simulink model "system_composer_test1"  (R2023b)
settings: Solver=VariableStepAuto  StartTime=0.0  StopTime=10.0  RelTol=1e-3
settings Model: Creator=jcm52  LastModifiedBy=jcm52

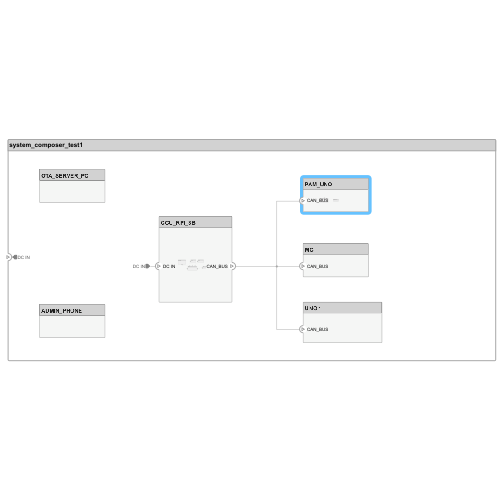
[thumbnail: Simulink's stored preview of the top-level diagram]
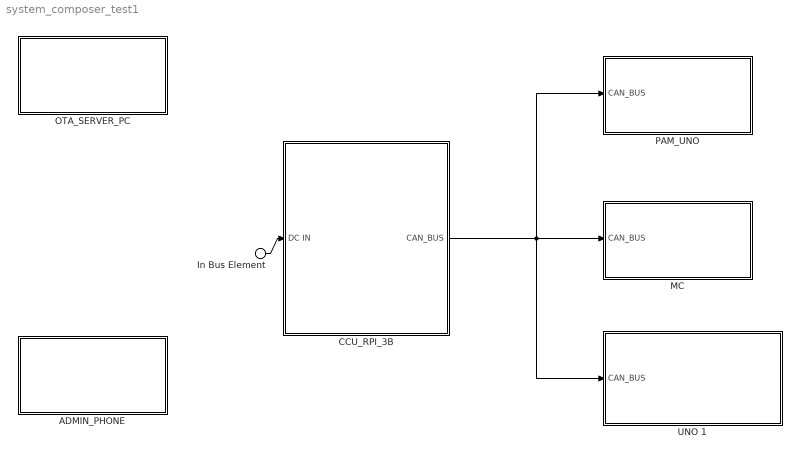
== system system_composer_test1 ==
  In Bus Element : Inport  PortName=DC IN
  ADMIN_PHONE : Subsystem
      settings: PortSchema="{\"entries\":[{\"content\":{\"headerSize\":26,\"margin\":15,\"minimumSpacing\":25,\"sides\":[{\"content\":{},\"type\":\"ConnectorPlacement.EquallySpacedRectSide\",\"uuid\":\"7e3d46c6-9eeb-4d23-9c3d-9bca39c5abc5\"},{\"content\":{\"side\":\"RIGHT\"},\"type\":\"ConnectorPlacement.EquallySpacedRectSide\",\"uuid\":\"9f2ff8fd-d14b-486f-a742-18e492795d25\"},{\"content\":{\"side\":\"TOP\"},\"type\":\"ConnectorPlacement.EquallySpacedRectSide\",\"uuid\":\"e95812f2-ccc1-4a86-ac53-e7b35601f911\"}]},\"type\":\"ConnectorPlacement.EquallySpacedConnector\",\"uuid\":\"2d0f1e9a-6af9-4d3f-b8da-a747a1ef6490\"}],\"packageUris\":[\"http://schema.mathworks.com/mf0/Connector/R2020b\"],\"version\":\"1.0\"}"
  CCU_RPI_3B : Subsystem
      settings: PortSchema="{\"entries\":[{\"content\":{\"headerSize\":26,\"margin\":15,\"minimumSpacing\":25,\"sides\":[{\"content\":{\"connectorIds\":[\"In1\"]},\"type\":\"ConnectorPlacement.EquallySpacedRectSide\",\"uuid\":\"35364ac4-dc3e-4266-bc20-925e01ca6202\"},{\"content\":{\"connectorIds\":[\"Out1\"],\"side\":\"RIGHT\"},\"type\":\"ConnectorPlacement.EquallySpacedRectSide\",\"uuid\":\"050ee6e0-40ef-4ced-bbf4-001a02d9c667\"},{\"content\":{\"side\":\"TOP\"},\"type\":\"ConnectorPlacement.EquallySpacedRectSide\",\"uuid\":\"0258bc82-266f-47dd-a28d-284b42f54e02\"},{\"content\":{\"side\":\"BOTTOM\"},\"type\":\"ConnectorPlacement.EquallySpacedRectSide\",\"uuid\":\"ceb5ff19-933f-4c7c-8606-80ebf5710174\"}]},\"type\":\"ConnectorPlacement.EquallySpacedConnector\",\"uuid\":\"a71d942b-361d-4a00-a580-c54bc0bd10ca\"}],\"packageUris\":[\"http://schema.mathworks.com/mf0/Connector/R2020b\"],\"version\":\"1.0\"}"
  MC : Subsystem
      settings: PortSchema="{\"entries\":[{\"content\":{\"headerSize\":26,\"margin\":15,\"minimumSpacing\":25,\"sides\":[{\"content\":{\"connectorIds\":[\"In1\"]},\"type\":\"ConnectorPlacement.EquallySpacedRectSide\",\"uuid\":\"35364ac4-dc3e-4266-bc20-925e01ca6202\"},{\"content\":{\"side\":\"RIGHT\"},\"type\":\"ConnectorPlacement.EquallySpacedRectSide\",\"uuid\":\"050ee6e0-40ef-4ced-bbf4-001a02d9c667\"},{\"content\":{\"side\":\"TOP\"},\"type\":\"ConnectorPlacement.EquallySpacedRectSide\",\"uuid\":\"0258bc82-266f-47dd-a28d-284b42f54e02\"}]},\"type\":\"ConnectorPlacement.EquallySpacedConnector\",\"uuid\":\"a71d942b-361d-4a00-a580-c54bc0bd10ca\"}],\"packageUris\":[\"http://schema.mathworks.com/mf0/Connector/R2020b\"],\"version\":\"1.0\"}"
  OTA_SERVER_PC : Subsystem
      settings: PortSchema="{\"entries\":[{\"content\":{\"headerSize\":26,\"margin\":15,\"minimumSpacing\":25,\"sides\":[{\"content\":{},\"type\":\"ConnectorPlacement.EquallySpacedRectSide\",\"uuid\":\"7e3d46c6-9eeb-4d23-9c3d-9bca39c5abc5\"},{\"content\":{\"side\":\"RIGHT\"},\"type\":\"ConnectorPlacement.EquallySpacedRectSide\",\"uuid\":\"9f2ff8fd-d14b-486f-a742-18e492795d25\"},{\"content\":{\"side\":\"TOP\"},\"type\":\"ConnectorPlacement.EquallySpacedRectSide\",\"uuid\":\"e95812f2-ccc1-4a86-ac53-e7b35601f911\"}]},\"type\":\"ConnectorPlacement.EquallySpacedConnector\",\"uuid\":\"2d0f1e9a-6af9-4d3f-b8da-a747a1ef6490\"}],\"packageUris\":[\"http://schema.mathworks.com/mf0/Connector/R2020b\"],\"version\":\"1.0\"}"
  PAM_UNO : Subsystem
      settings: PortSchema="{\"entries\":[{\"content\":{\"headerSize\":26,\"margin\":15,\"minimumSpacing\":25,\"sides\":[{\"content\":{\"connectorIds\":[\"In1\"]},\"type\":\"ConnectorPlacement.EquallySpacedRectSide\",\"uuid\":\"35364ac4-dc3e-4266-bc20-925e01ca6202\"},{\"content\":{\"side\":\"RIGHT\"},\"type\":\"ConnectorPlacement.EquallySpacedRectSide\",\"uuid\":\"050ee6e0-40ef-4ced-bbf4-001a02d9c667\"},{\"content\":{\"side\":\"TOP\"},\"type\":\"ConnectorPlacement.EquallySpacedRectSide\",\"uuid\":\"0258bc82-266f-47dd-a28d-284b42f54e02\"}]},\"type\":\"ConnectorPlacement.EquallySpacedConnector\",\"uuid\":\"a71d942b-361d-4a00-a580-c54bc0bd10ca\"}],\"packageUris\":[\"http://schema.mathworks.com/mf0/Connector/R2020b\"],\"version\":\"1.0\"}"
  UNO 1 : Subsystem
      settings: PortSchema="{\"entries\":[{\"content\":{\"headerSize\":26,\"margin\":15,\"minimumSpacing\":25,\"sides\":[{\"content\":{\"connectorIds\":[\"In1\"]},\"type\":\"ConnectorPlacement.EquallySpacedRectSide\",\"uuid\":\"35364ac4-dc3e-4266-bc20-925e01ca6202\"},{\"content\":{\"side\":\"RIGHT\"},\"type\":\"ConnectorPlacement.EquallySpacedRectSide\",\"uuid\":\"050ee6e0-40ef-4ced-bbf4-001a02d9c667\"},{\"content\":{\"side\":\"TOP\"},\"type\":\"ConnectorPlacement.EquallySpacedRectSide\",\"uuid\":\"0258bc82-266f-47dd-a28d-284b42f54e02\"}]},\"type\":\"ConnectorPlacement.EquallySpacedConnector\",\"uuid\":\"a71d942b-361d-4a00-a580-c54bc0bd10ca\"}],\"packageUris\":[\"http://schema.mathworks.com/mf0/Connector/R2020b\"],\"version\":\"1.0\"}"
  wires:
  In Bus Element/1 -> CCU_RPI_3B/1(DC IN)
  CCU_RPI_3B/1(CAN_BUS) -> UNO 1/1(CAN_BUS), PAM_UNO/1(CAN_BUS), MC/1(CAN_BUS)

== system system_composer_test1/ADMIN_PHONE ==

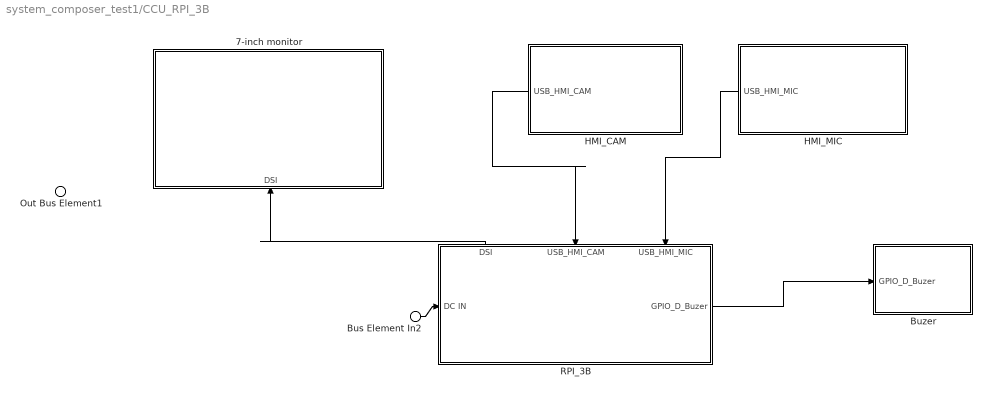
== system system_composer_test1/CCU_RPI_3B ==
  Bus Element In2 : Inport  PortName=DC IN
  7-inch monitor : Subsystem
      settings: PortSchema="{\"entries\":[{\"content\":{\"headerSize\":26,\"margin\":15,\"minimumSpacing\":25,\"sides\":[{\"content\":{},\"type\":\"ConnectorPlacement.EquallySpacedRectSide\",\"uuid\":\"35364ac4-dc3e-4266-bc20-925e01ca6202\"},{\"content\":{\"side\":\"RIGHT\"},\"type\":\"ConnectorPlacement.EquallySpacedRectSide\",\"uuid\":\"050ee6e0-40ef-4ced-bbf4-001a02d9c667\"},{\"content\":{\"side\":\"TOP\"},\"type\":\"ConnectorPlacement.EquallySpacedRectSide\",\"uuid\":\"0258bc82-266f-47dd-a28d-284b42f54e02\"},{\"content\":{\"connectorIds\":[\"In1\"],\"side\":\"BOTTOM\"},\"type\":\"ConnectorPlacement.EquallySpacedRectSide\",\"uuid\":\"164fd1d1-7818-47b7-85b0-d89fae4b1f16\"}]},\"type\":\"ConnectorPlacement.EquallySpacedConnector\",\"uuid\":\"a71d942b-361d-4a00-a580-c54bc0bd10ca\"}],\"packageUris\":[\"http://schema.mathworks.com/mf0/Connector/R2020b\"],\"version\":\"1.0\"}"
  Buzer : Subsystem
      settings: PortSchema="{\"entries\":[{\"content\":{\"headerSize\":26,\"margin\":15,\"minimumSpacing\":25,\"sides\":[{\"content\":{\"connectorIds\":[\"In1\"]},\"type\":\"ConnectorPlacement.EquallySpacedRectSide\",\"uuid\":\"7e3d46c6-9eeb-4d23-9c3d-9bca39c5abc5\"},{\"content\":{\"side\":\"RIGHT\"},\"type\":\"ConnectorPlacement.EquallySpacedRectSide\",\"uuid\":\"9f2ff8fd-d14b-486f-a742-18e492795d25\"},{\"content\":{\"side\":\"TOP\"},\"type\":\"ConnectorPlacement.EquallySpacedRectSide\",\"uuid\":\"e95812f2-ccc1-4a86-ac53-e7b35601f911\"}]},\"type\":\"ConnectorPlacement.EquallySpacedConnector\",\"uuid\":\"2d0f1e9a-6af9-4d3f-b8da-a747a1ef6490\"}],\"packageUris\":[\"http://schema.mathworks.com/mf0/Connector/R2020b\"],\"version\":\"1.0\"}"
  HMI_CAM : Subsystem
      settings: PortSchema="{\"entries\":[{\"content\":{\"headerSize\":26,\"margin\":15,\"minimumSpacing\":25,\"sides\":[{\"content\":{\"connectorIds\":[\"Out1\"]},\"type\":\"ConnectorPlacement.EquallySpacedRectSide\",\"uuid\":\"35364ac4-dc3e-4266-bc20-925e01ca6202\"},{\"content\":{\"side\":\"RIGHT\"},\"type\":\"ConnectorPlacement.EquallySpacedRectSide\",\"uuid\":\"050ee6e0-40ef-4ced-bbf4-001a02d9c667\"},{\"content\":{\"side\":\"TOP\"},\"type\":\"ConnectorPlacement.EquallySpacedRectSide\",\"uuid\":\"0258bc82-266f-47dd-a28d-284b42f54e02\"}]},\"type\":\"ConnectorPlacement.EquallySpacedConnector\",\"uuid\":\"a71d942b-361d-4a00-a580-c54bc0bd10ca\"}],\"packageUris\":[\"http://schema.mathworks.com/mf0/Connector/R2020b\"],\"version\":\"1.0\"}"
  HMI_MIC : Subsystem
      settings: PortSchema="{\"entries\":[{\"content\":{\"headerSize\":26,\"margin\":15,\"minimumSpacing\":25,\"sides\":[{\"content\":{\"connectorIds\":[\"Out1\"]},\"type\":\"ConnectorPlacement.EquallySpacedRectSide\",\"uuid\":\"7e3d46c6-9eeb-4d23-9c3d-9bca39c5abc5\"},{\"content\":{\"side\":\"RIGHT\"},\"type\":\"ConnectorPlacement.EquallySpacedRectSide\",\"uuid\":\"9f2ff8fd-d14b-486f-a742-18e492795d25\"},{\"content\":{\"side\":\"TOP\"},\"type\":\"ConnectorPlacement.EquallySpacedRectSide\",\"uuid\":\"e95812f2-ccc1-4a86-ac53-e7b35601f911\"}]},\"type\":\"ConnectorPlacement.EquallySpacedConnector\",\"uuid\":\"2d0f1e9a-6af9-4d3f-b8da-a747a1ef6490\"}],\"packageUris\":[\"http://schema.mathworks.com/mf0/Connector/R2020b\"],\"version\":\"1.0\"}"
  RPI_3B : Subsystem
      settings: PortSchema="{\"entries\":[{\"content\":{\"headerSize\":26,\"margin\":15,\"minimumSpacing\":25,\"sides\":[{\"content\":{\"connectorIds\":[\"In1\"]},\"type\":\"ConnectorPlacement.EquallySpacedRectSide\",\"uuid\":\"7e3d46c6-9eeb-4d23-9c3d-9bca39c5abc5\"},{\"content\":{\"connectorIds\":[\"Out1\"],\"side\":\"RIGHT\"},\"type\":\"ConnectorPlacement.EquallySpacedRectSide\",\"uuid\":\"9f2ff8fd-d14b-486f-a742-18e492795d25\"},{\"content\":{\"connectorIds\":[\"Out2\",\"In2\",\"In3\"],\"side\":\"TOP\"},\"type\":\"ConnectorPlacement.EquallySpacedRectSide\",\"uuid\":\"e95812f2-ccc1-4a86-ac53-e7b35601f911\"}]},\"type\":\"ConnectorPlacement.EquallySpacedConnector\",\"uuid\":\"2d0f1e9a-6af9-4d3f-b8da-a747a1ef6490\"}],\"packageUris\":[\"http://schema.mathworks.com/mf0/Connector/R2020b\"],\"version\":\"1.0\"}"
  Out Bus Element1 : Outport  PortName=CAN_BUS
  wires:
  HMI_CAM/1(USB_HMI_CAM) -> RPI_3B/2(USB_HMI_CAM)
  HMI_MIC/1(USB_HMI_MIC) -> RPI_3B/3(USB_HMI_MIC)
  RPI_3B/2(DSI) -> 7-inch monitor/1(DSI)
  Bus Element In2/1 -> RPI_3B/1(DC IN)
  RPI_3B/1(GPIO_D_Buzer) -> Buzer/1(GPIO_D_Buzer)

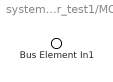
== system system_composer_test1/MC ==
  Bus Element In1 : Inport  PortName=CAN_BUS

== system system_composer_test1/OTA_SERVER_PC ==

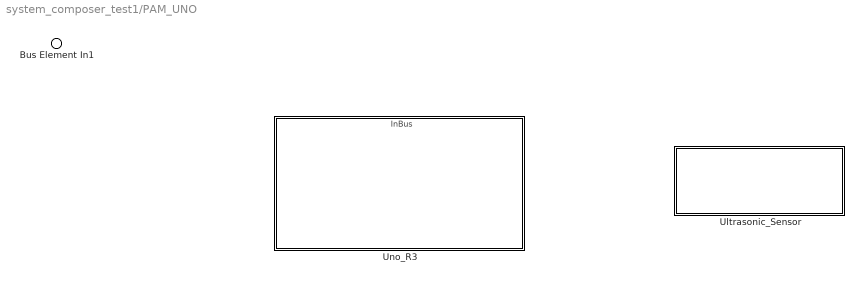
== system system_composer_test1/PAM_UNO ==
  Bus Element In1 : Inport  PortName=CAN_BUS
  Ultrasonic_Sensor : Subsystem
      settings: PortSchema="{\"entries\":[{\"content\":{\"headerSize\":26,\"margin\":15,\"minimumSpacing\":25,\"sides\":[{\"content\":{},\"type\":\"ConnectorPlacement.EquallySpacedRectSide\",\"uuid\":\"7e3d46c6-9eeb-4d23-9c3d-9bca39c5abc5\"},{\"content\":{\"side\":\"RIGHT\"},\"type\":\"ConnectorPlacement.EquallySpacedRectSide\",\"uuid\":\"9f2ff8fd-d14b-486f-a742-18e492795d25\"},{\"content\":{\"side\":\"TOP\"},\"type\":\"ConnectorPlacement.EquallySpacedRectSide\",\"uuid\":\"e95812f2-ccc1-4a86-ac53-e7b35601f911\"}]},\"type\":\"ConnectorPlacement.EquallySpacedConnector\",\"uuid\":\"2d0f1e9a-6af9-4d3f-b8da-a747a1ef6490\"}],\"packageUris\":[\"http://schema.mathworks.com/mf0/Connector/R2020b\"],\"version\":\"1.0\"}"
  Uno_R3 : Subsystem
      settings: PortSchema="{\"entries\":[{\"content\":{\"headerSize\":26,\"margin\":15,\"minimumSpacing\":25,\"sides\":[{\"content\":{},\"type\":\"ConnectorPlacement.EquallySpacedRectSide\",\"uuid\":\"7e3d46c6-9eeb-4d23-9c3d-9bca39c5abc5\"},{\"content\":{\"side\":\"RIGHT\"},\"type\":\"ConnectorPlacement.EquallySpacedRectSide\",\"uuid\":\"9f2ff8fd-d14b-486f-a742-18e492795d25\"},{\"content\":{\"connectorIds\":[\"In1\"],\"side\":\"TOP\"},\"type\":\"ConnectorPlacement.EquallySpacedRectSide\",\"uuid\":\"e95812f2-ccc1-4a86-ac53-e7b35601f911\"}]},\"type\":\"ConnectorPlacement.EquallySpacedConnector\",\"uuid\":\"2d0f1e9a-6af9-4d3f-b8da-a747a1ef6490\"}],\"packageUris\":[\"http://schema.mathworks.com/mf0/Connector/R2020b\"],\"version\":\"1.0\"}"

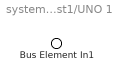
== system system_composer_test1/UNO 1 ==
  Bus Element In1 : Inport  PortName=CAN_BUS

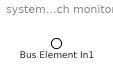
== system system_composer_test1/CCU_RPI_3B/7-inch monitor ==
  Bus Element In1 : Inport  PortName=DSI

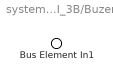
== system system_composer_test1/CCU_RPI_3B/Buzer ==
  Bus Element In1 : Inport  PortName=GPIO_D_Buzer

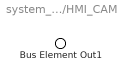
== system system_composer_test1/CCU_RPI_3B/HMI_CAM ==
  Bus Element Out1 : Outport  PortName=USB_HMI_CAM

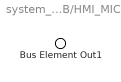
== system system_composer_test1/CCU_RPI_3B/HMI_MIC ==
  Bus Element Out1 : Outport  PortName=USB_HMI_MIC

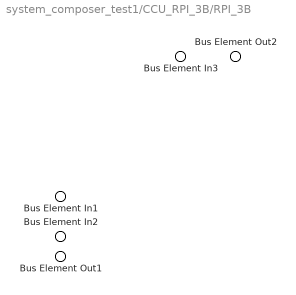
== system system_composer_test1/CCU_RPI_3B/RPI_3B ==
  Bus Element In3 : Inport  PortName=DC IN
  Bus Element In1 : Inport  Port=2  PortName=USB_HMI_CAM
  Bus Element In2 : Inport  Port=3  PortName=USB_HMI_MIC
  Bus Element Out2 : Outport  PortName=GPIO_D_Buzer
  Bus Element Out1 : Outport  Port=2  PortName=DSI

== system system_composer_test1/PAM_UNO/Ultrasonic_Sensor ==

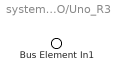
== system system_composer_test1/PAM_UNO/Uno_R3 ==
  Bus Element In1 : Inport  PortName=InBus
